simulink model "MBD_Sources_Input"  (R2021b)
settings: Solver=FixedStepDiscrete  StartTime=0.0  StopTime=10.0  RelTol=1e-3
settings Model: Creator=waleed.elshemy  LastModifiedBy=waleed.elshemy

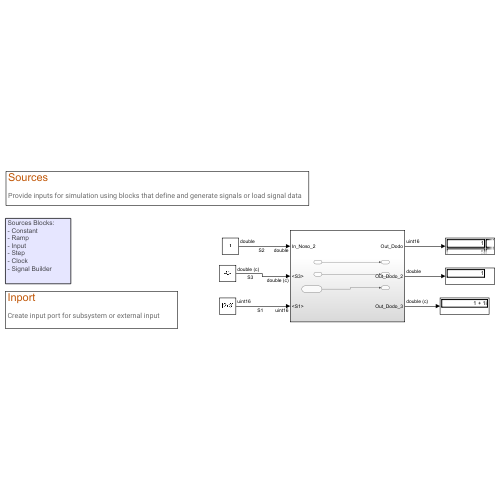
[thumbnail: Simulink's stored preview of the top-level diagram]
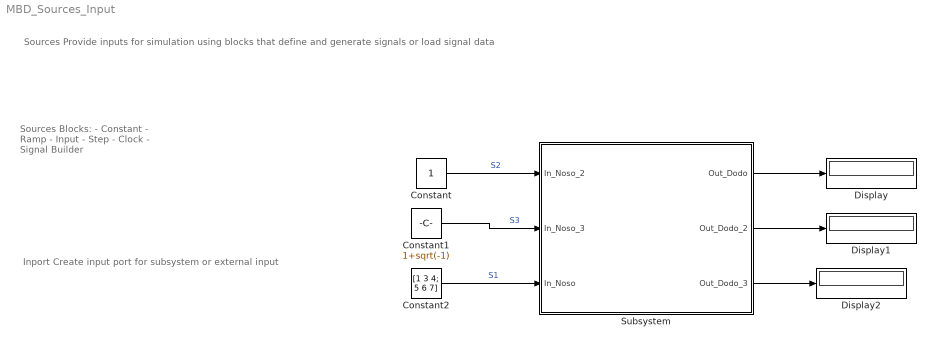
== system MBD_Sources_Input ==
  note: Inport
      | Create input port for subsystem or external input
  note: Sources
      | Provide inputs for simulation using blocks that define and generate signals or load signal data
  note: Sources Blocks:
      | - Constant
      | - Ramp
      | - Input
      | - Step
      | - Clock
      | - Signal Builder
  Constant : Constant
  Constant1 : Constant  Value=1+sqrt(-1)
  Constant2 : Constant  Value=[1 3 4; 5 6 7]  OutDataTypeStr=uint16
  Display : Display
  Display1 : Display
  Display2 : Display
  Subsystem : Subsystem
  wires:
  Constant/1 -> Subsystem/1(In_Noso_2)  "S2"
  Constant1/1 -> Subsystem/2(In_Noso_3)  "S3"
  Constant2/1 -> Subsystem/3(In_Noso)  "S1"
  Subsystem/1(Out_Dodo) -> Display/1
  Subsystem/2(Out_Dodo_2) -> Display1/1
  Subsystem/3(Out_Dodo_3) -> Display2/1

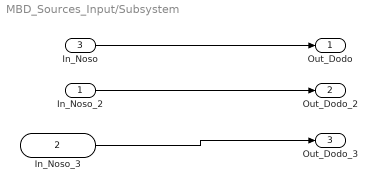
== system MBD_Sources_Input/Subsystem ==
  In_Noso_2 : Inport
  In_Noso_3 : Inport  Port=2
      settings: SignalType=complex
  In_Noso : Inport  Port=3  OutDataTypeStr=uint16  PortDimensions=[2 3]
  Out_Dodo : Outport
  Out_Dodo_2 : Outport  Port=2
  Out_Dodo_3 : Outport  Port=3
  wires:
  In_Noso/1 -> Out_Dodo/1
  In_Noso_2/1 -> Out_Dodo_2/1
  In_Noso_3/1 -> Out_Dodo_3/1
